simulink model "levitatore"  (R2017a)
settings: Solver=VariableStepAuto  StartTime=0.0  StopTime=2  RelTol=1e-3
values from neighbouring files (symbols this model uses):
  b = 0.1    [levitatoreMagnetico.m]    (also in temp1.mat)
  g = 9.81    [levitatoreMagnetico.m]    (also in temp1.mat)
  km = 19.62    [levitatoreMagnetico.m]    (also in temp1.mat)
  L0 = 0.5    [levitatoreMagnetico.m]    (also in temp1.mat)
  m = 0.2    [levitatoreMagnetico.m]    (also in temp1.mat)
  R = 50    [levitatoreMagnetico.m]    (also in temp1.mat)
  ueq = 5    [levitatoreMagnetico.m]    (also in temp1.mat)
settings Model: Creator=Enrico Donato  LastModifiedBy=Enrico Donato

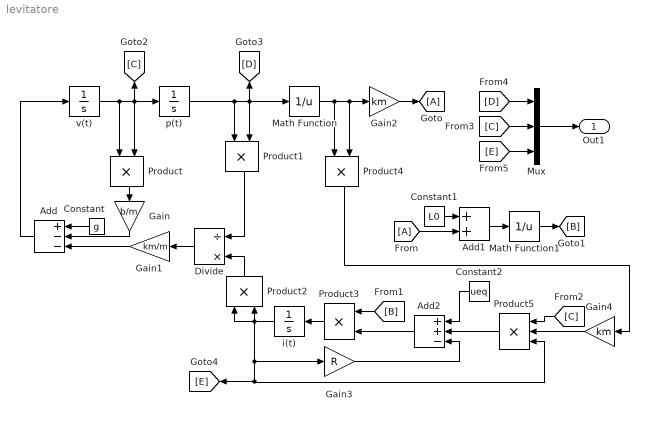
== system levitatore ==
  Add : Sum  Inputs=+--
  Add1 : Sum
  Add2 : Sum  Inputs=++-
  Constant : Constant  Value=g
  Constant1 : Constant  Value=L0
  Constant2 : Constant  Value=ueq
  Divide : Product  Inputs=/*
  Gain : Gain  Gain=b/m
  Gain1 : Gain  Gain=km/m
  Gain2 : Gain  Gain=km
  Gain3 : Gain  Gain=R
  Gain4 : Gain  Gain=km
  Math Function : Math  Operator=reciprocal  SaturateOnIntegerOverflow=on
  Math Function1 : Math  Operator=reciprocal  SaturateOnIntegerOverflow=on
  Mux : Mux  Inputs=3
  Product{,1..4} (5 alike) : Product
  Product5 : Product  Inputs=3
  i(t) : Integrator
  p(t) : Integrator
  v(t) : Integrator
  Out1 : Outport  SignalName=x(t)
  wires:
  v(t)/1 -> Product/1, p(t)/1, [C], Product/2
  Constant/1 -> Add/1
  Product/1 -> Gain/1
  Gain/1 -> Add/2
  Gain1/1 -> Add/3
  Product1/1 -> Divide/1
  Divide/1 -> Gain1/1
  Product2/1 -> Divide/2
  i(t)/1 -> Product5/3, [E], Gain3/1, Product2/1, Product2/2
  Add/1 -> v(t)/1
  Constant1/1 -> Add1/1
  Math Function/1 -> Product4/1, Product4/2, Gain2/1
  [A] -> Add1/2
  Add1/1 -> Math Function1/1
  Math Function1/1 -> [B]
  Product3/1 -> i(t)/1
  [B] -> Product3/1
  Add2/1 -> Product3/2
  Gain3/1 -> Add2/3
  Gain2/1 -> [A]
  Product5/1 -> Add2/2
  [C] -> Product5/1
  Product4/1 -> Gain4/1
  Gain4/1 -> Product5/2
  Mux/1 -> Out1/1
  [C] -> Mux/2
  [E] -> Mux/3
  p(t)/1 -> [D], Math Function/1, Product1/2, Product1/1
  [D] -> Mux/1
  Constant2/1 -> Add2/1
